simulink model "Daniela_impedance_matching_position_force_compensation"  (R2016a)
settings: Solver=ode45  StartTime=0.0  StopTime=30  RelTol=1e-3
values from neighbouring files (symbols this model uses):
  b = 5    [Daniela_basic_parameters.m]    (also in Tanner_Niemeyer_high_frequency_force_parameters.m = 2.5; Tanner_Niemeyer_wave_filtering_parameters.m = 2.5; Xizhe_wave_filtering_parameters.m = 300; Ye_Liu_augmented_trajectory_tracking_parameters.m = 2.5)
  bm = 0.005    [Daniela_basic_parameters.m]    (also in Tanner_Niemeyer_high_frequency_force_parameters.m; Tanner_Niemeyer_wave_filtering_parameters.m; Xizhe_wave_filtering_parameters.m; Ye_Liu_augmented_trajectory_tracking_parameters.m = 2.5)
  bs = 0.005    [Daniela_basic_parameters.m]    (also in Tanner_Niemeyer_high_frequency_force_parameters.m; Tanner_Niemeyer_wave_filtering_parameters.m; Xizhe_wave_filtering_parameters.m; Ye_Liu_augmented_trajectory_tracking_parameters.m = 2.5)
  Jm = 1    [Daniela_basic_parameters.m]    (also in Tanner_Niemeyer_high_frequency_force_parameters.m = 0.1; Tanner_Niemeyer_wave_filtering_parameters.m = 0.1; Xizhe_wave_filtering_parameters.m; Ye_Liu_augmented_trajectory_tracking_parameters.m = 0.1)
  Js = 1    [Daniela_basic_parameters.m]    (also in Tanner_Niemeyer_high_frequency_force_parameters.m = 0.1; Tanner_Niemeyer_wave_filtering_parameters.m = 0.1; Xizhe_wave_filtering_parameters.m; Ye_Liu_augmented_trajectory_tracking_parameters.m = 0.1)
  Ki = 200    [Daniela_basic_parameters.m]    (also in Tanner_Niemeyer_high_frequency_force_parameters.m = 370; Tanner_Niemeyer_wave_filtering_parameters.m = 370; Xizhe_wave_filtering_parameters.m = 2000; Ye_Liu_augmented_trajectory_tracking_parameters.m = 370)
  Kp = 1    [Daniela_basic_parameters.m]    (also in Tanner_Niemeyer_high_frequency_force_parameters.m = 2.5; Tanner_Niemeyer_wave_filtering_parameters.m = 2.5; Xizhe_wave_filtering_parameters.m = 200; Ye_Liu_augmented_trajectory_tracking_parameters.m = 20)
  Td = 0.03    [Daniela_basic_parameters.m]    (also in Tanner_Niemeyer_high_frequency_force_parameters.m; Tanner_Niemeyer_wave_filtering_parameters.m = 0.1; Xizhe_wave_filtering_parameters.m; Ye_Liu_augmented_trajectory_tracking_parameters.m = 0.5)
  x_m0 = 0    [Daniela_basic_parameters.m]    (also in Tanner_Niemeyer_high_frequency_force_parameters.m; Tanner_Niemeyer_wave_filtering_parameters.m; Xizhe_wave_filtering_parameters.m; Ye_Liu_augmented_trajectory_tracking_parameters.m)
  x_s0 = 0    [Daniela_basic_parameters.m]    (also in Tanner_Niemeyer_high_frequency_force_parameters.m; Tanner_Niemeyer_wave_filtering_parameters.m; Xizhe_wave_filtering_parameters.m; Ye_Liu_augmented_trajectory_tracking_parameters.m)
  xdot_m0 = 0    [Daniela_basic_parameters.m]    (also in Tanner_Niemeyer_high_frequency_force_parameters.m; Tanner_Niemeyer_wave_filtering_parameters.m; Xizhe_wave_filtering_parameters.m; Ye_Liu_augmented_trajectory_tracking_parameters.m)
  xdot_s0 = 0    [Daniela_basic_parameters.m]    (also in Tanner_Niemeyer_high_frequency_force_parameters.m; Tanner_Niemeyer_wave_filtering_parameters.m; Xizhe_wave_filtering_parameters.m; Ye_Liu_augmented_trajectory_tracking_parameters.m)
libraries: simulink x1
settings Model: Creator=Administrator  LastModifiedBy=sunxizhe
settings HardwareCC: ProdWordSize=32  ProdHWDeviceType=Specified

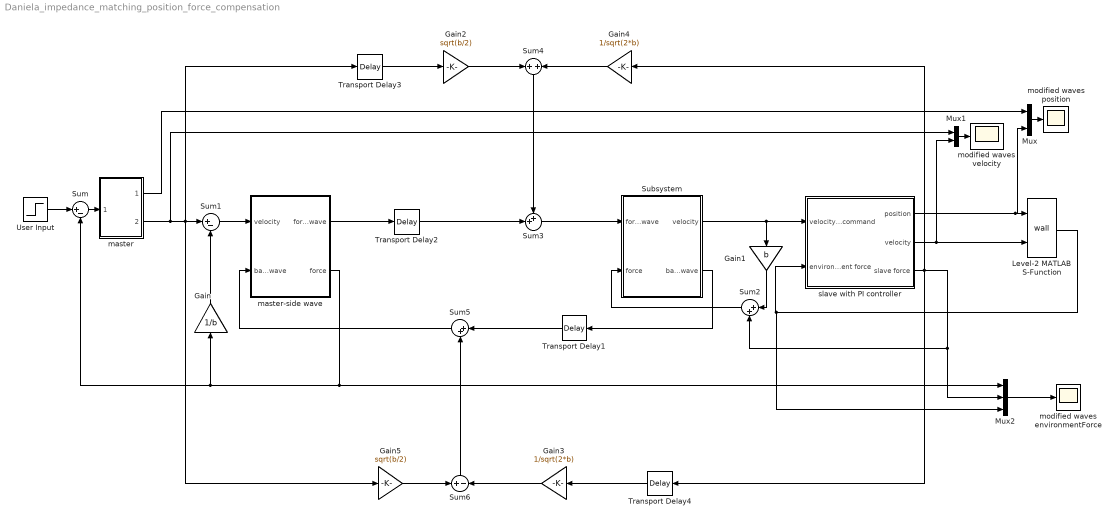
== system Daniela_impedance_matching_position_force_compensation ==
  Gain : Gain  Gain=1/b
  Gain1 : Gain  Gain=b
  Gain2 : Gain  Gain=sqrt(b/2)
  Gain3 : Gain  Gain=1/sqrt(2*b)
  Gain4 : Gain  Gain=1/sqrt(2*b)
  Gain5 : Gain  Gain=sqrt(b/2)
  Level-2 MATLAB S-Function : M-S-Function  FunctionName=wall  Parameters=Kwall, bwall, xwall
  Mux : Mux  Inputs=2
  Mux1 : Mux  Inputs=2
  Mux2 : Mux  Inputs=3
  Subsystem : Subsystem
  Sum : Sum  Inputs=|+-
  Sum1 : Sum  Inputs=|+-
  Sum2 : Sum  Inputs=|++
  Sum3 : Sum  Inputs=++|
  Sum4 : Sum  Inputs=+|+
  Sum5 : Sum  Inputs=|++
  Sum6 : Sum  Inputs=+|-
  Transport Delay{1..4} (4 alike) : TransportDelay  DelayTime=Td
  User Input : Step  Time=0  SampleTime=0
  "master " : Subsystem
  master-side wave : Subsystem
  modified waves environmentForce : Scope
  modified waves position : Scope
  modified waves velocity : Scope
  slave with PI controller : Subsystem
  wires:
  Level-2 MATLAB S-Function/1 -> slave with PI controller/2(environment force), Mux2/3
  Mux/1 -> modified waves position/1
  master-side wave/2(force) -> Mux2/1, Sum/2, Gain/1
  master-side wave/1(forward wave) -> Transport Delay2/1
  Subsystem/2(backward wave) -> Transport Delay1/1
  "master "/1("position ") -> Mux/1
  Sum/1 -> "master "/1(force)
  slave with PI controller/1(position) -> Level-2 MATLAB S-Function/1, Mux/2
  slave with PI controller/2(velocity) -> Level-2 MATLAB S-Function/2, Mux1/2
  slave with PI controller/3(slave force) -> Transport Delay4/1, Gain4/1, Sum2/2, Mux2/2
  Mux2/1 -> modified waves environmentForce/1
  Sum1/1 -> master-side wave/1(velocity)
  "master "/2(velocity) -> Mux1/1, Sum1/1, Gain5/1, Transport Delay3/1
  Sum2/1 -> Subsystem/2(force)
  Subsystem/1(velocity) -> Gain1/1, slave with PI controller/1(velocity command)
  Mux1/1 -> modified waves velocity/1
  User Input/1 -> Sum/1
  Gain1/1 -> Sum2/1
  Gain/1 -> Sum1/2
  Transport Delay3/1 -> Gain2/1
  Gain2/1 -> Sum4/1
  Gain4/1 -> Sum4/2
  Sum3/1 -> Subsystem/1(forward wave)
  Transport Delay2/1 -> Sum3/2
  Sum4/1 -> Sum3/1
  Transport Delay1/1 -> Sum5/1
  Sum5/1 -> master-side wave/2(backward wave)
  Gain5/1 -> Sum6/1
  Gain3/1 -> Sum6/2
  Transport Delay4/1 -> Gain3/1
  Sum6/1 -> Sum5/2

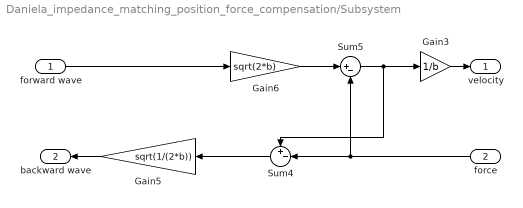
== system Daniela_impedance_matching_position_force_compensation/Subsystem ==
  forward wave : Inport
  force : Inport  Port=2
  Gain3 : Gain  Gain=1/b
  Gain5 : Gain  Gain=sqrt(1/(2*b))
  Gain6 : Gain  Gain=sqrt(2*b)
  Sum4 : Sum  Inputs=+-|
  Sum5 : Sum  Inputs=|+-
  velocity : Outport
  backward wave : Outport  Port=2
  wires:
  forward wave/1 -> Gain6/1
  Gain6/1 -> Sum5/1
  Sum5/1 -> Sum4/1, Gain3/1
  Gain3/1 -> velocity/1
  Gain5/1 -> backward wave/1
  Sum4/1 -> Gain5/1
  force/1 -> Sum4/2, Sum5/2

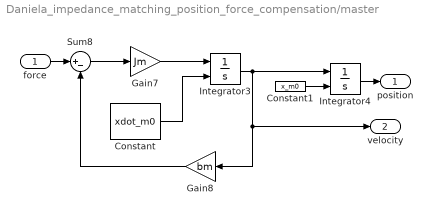
== system Daniela_impedance_matching_position_force_compensation/master  ==
  force : Inport
  Constant : Constant  Value=xdot_m0
  Constant1 : Constant  Value=x_m0
  Gain7 : Gain  Gain=Jm
  Gain8 : Gain  Gain=bm
  Integrator3 : Integrator  InitialConditionSource=external
  Integrator4 : Integrator  InitialConditionSource=external
  Sum8 : Sum  Inputs=|+-
  "position " : Outport
  velocity : Outport  Port=2
  wires:
  Integrator3/1 -> Integrator4/1, velocity/1, Gain8/1
  Sum8/1 -> Gain7/1
  Gain8/1 -> Sum8/2
  force/1 -> Sum8/1
  Integrator4/1 -> "position "/1
  Constant/1 -> Integrator3/2
  Constant1/1 -> Integrator4/2
  Gain7/1 -> Integrator3/1

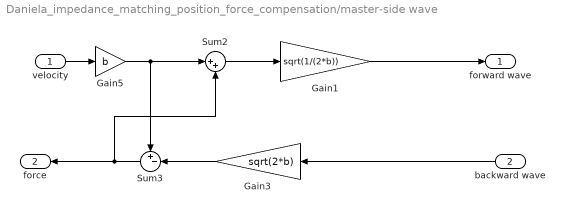
== system Daniela_impedance_matching_position_force_compensation/master-side wave ==
  velocity : Inport
  backward wave : Inport  Port=2
  Gain1 : Gain  Gain=sqrt(1/(2*b))
  Gain3 : Gain  Gain=sqrt(2*b)
  Gain5 : Gain  Gain=b
  Sum2 : Sum  Inputs=|++
  Sum3 : Sum  Inputs=+-|
  forward wave : Outport
  force : Outport  Port=2
  wires:
  Sum3/1 -> Sum2/2, force/1
  backward wave/1 -> Gain3/1
  Gain1/1 -> forward wave/1
  Gain3/1 -> Sum3/2
  velocity/1 -> Gain5/1
  Sum2/1 -> Gain1/1
  Gain5/1 -> Sum3/1, Sum2/1

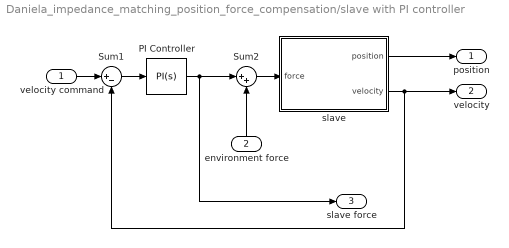
== system Daniela_impedance_matching_position_force_compensation/slave with PI controller ==
  velocity command : Inport
  environment force : Inport  Port=2
  PI Controller : simulink/Continuous/PID Controller  Controller=PI  TimeDomain=Continuous-time  SampleTime=-1  IntegratorMethod=Forward Euler  FilterMethod=Forward Euler  Form=Parallel  UseFilter=on  ControllerParametersSource=internal  P=Kp  I=Ki  D=0  N=100  InitialConditionSource=internal  InitialConditionForIntegrator=0  InitialConditionForFilter=0  ExternalReset=none  LimitOutput=off  UpperSaturationLimit=inf  LowerSaturationLimit=-inf  LinearizeAsGain=on  AntiWindupMode=none  Kb=1  TrackingMode=off  Kt=1  PParamMin=[]  PParamMax=[]  IParamMin=[]  IParamMax=[]  DParamMin=[]  DParamMax=[]  NParamMin=[]  NParamMax=[]  KbParamMin=[]  KbParamMax=[]  KtParamMin=[]  KtParamMax=[]  POutMin=[]  POutMax=[]  IOutMin=[]  IOutMax=[]  DOutMin=[]  DOutMax=[]  NOutMin=[]  NOutMax=[]  KbOutMin=[]  KbOutMax=[]  KtOutMin=[]  KtOutMax=[]  IntegratorOutMin=[]  IntegratorOutMax=[]  FilterOutMin=[]  FilterOutMax=[]  SumOutMin=[]  SumOutMax=[]  SumI1OutMin=[]  SumI1OutMax=[]  SumI2OutMin=[]  SumI2OutMax=[]  SumI3OutMin=[]  SumI3OutMax=[]  SumDOutMin=[]  SumDOutMax=[]  SaturationOutMin=[]  SaturationOutMax=[]  IntegratorContinuousStateAttributes=''  IntegratorStateMustResolveToSignalObject=off  IntegratorRTWStateStorageClass=Auto  FilterContinuousStateAttributes=''  FilterStateMustResolveToSignalObject=off  FilterRTWStateStorageClass=Auto  DifferentiatorICPrevScaledInput=0  DifferentiatorOutMin=[]  DifferentiatorOutMax=[]
  Sum1 : Sum  Inputs=|+-
  Sum2 : Sum  Inputs=|++
  "slave " : Subsystem
  position : Outport
  velocity : Outport  Port=2
  slave force : Outport  Port=3
  wires:
  Sum1/1 -> PI Controller/1
  "slave "/1("position ") -> position/1
  environment force/1 -> Sum2/2
  PI Controller/1 -> slave force/1, Sum2/1
  Sum2/1 -> "slave "/1(force)
  velocity command/1 -> Sum1/1
  "slave "/2(velocity) -> velocity/1, Sum1/2

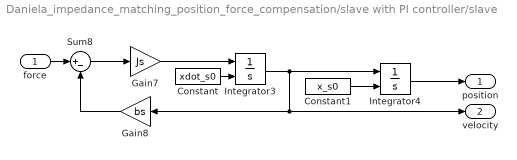
== system Daniela_impedance_matching_position_force_compensation/slave with PI controller/slave  ==
  force : Inport
  Constant : Constant  Value=xdot_s0
  Constant1 : Constant  Value=x_s0
  Gain7 : Gain  Gain=Js
  Gain8 : Gain  Gain=bs
  Integrator3 : Integrator  InitialConditionSource=external
  Integrator4 : Integrator  InitialConditionSource=external
  Sum8 : Sum  Inputs=|+-
  "position " : Outport
  velocity : Outport  Port=2
  wires:
  Integrator3/1 -> Integrator4/1, Gain8/1, velocity/1
  Sum8/1 -> Gain7/1
  Gain8/1 -> Sum8/2
  force/1 -> Sum8/1
  Integrator4/1 -> "position "/1
  Constant/1 -> Integrator3/2
  Gain7/1 -> Integrator3/1
  Constant1/1 -> Integrator4/2
